simulink model "Engine_MvMdl_Ptbs_V1"  (R2018a)
settings: Solver=VariableStepAuto  StartTime=0.0  StopTime=660  FixedStep=0.001  EnableMultiTasking=on
PreLoadFcn:
  | Engine_MapMdl_Ptbs_V1_BusInfo
model workspace (MAT data in the model file):
  DiffRatio = 3.421
  EV_current = 200
  EV_motion = [20 4 0.8]
  EV_sf = 2000
  EngDriveRatio = 0.813008130081
  Fs = 0
  Fv = 0.0025
  Jcomp = 0.0227
  Jengine = 0.22
  Ki = 251.3274
  Kisa = 346.6583
  Kp_d = 0.47149
  Kp_q = 0.52125
  Ksa = 85.4316
  Ksf = 1996.2651
  Ld = 0.0003752
  Ldq = [0.0003752 0.0004148]
  Lq = 0.0004148
  Mechanical = [0.0227 0.0025 0]
  MotGbRatio = 1
  P = 4
  PolePairs = 4
  RWheel = 0.3
  Rs = 0.2
  T_max = 120
  T_mtpa = [0 13.3131834767 26.6278836885 39.9456159322 53.2678926341 66.5962219318 79.9321062746 93.277041051 106.632513247 120.000000141]
  b_axle = Simulink.Parameter
  b_axle.Value = 10
  b_axle.DataType = 'auto'
  b_axle.Dimensions = [1 1]
  b_driveshaft = Simulink.Parameter
  b_driveshaft.Value = 10
  b_driveshaft.DataType = 'auto'
  b_driveshaft.Dimensions = [1 1]
  ba = 3.4029
  id_mtpa = [0 -0.114523352646 -0.457989076459 -1.03008464374 -1.83029075221 -2.85788367342 -4.11193850568 -5.59133329791 -7.29475400168 -9.22070020138]
  idq0 = [0 0]
  idq_limits = [-9.220699542 166.993501392 167.247872355]
  iq_mtpa = [0 18.5827440345 37.1633719111 55.7397734896 74.3098506185 92.871523015 111.422734008 129.961456105 148.485696337 166.993501356]
  k_axle = Simulink.Parameter
  k_axle.Value = 5000
  k_axle.DataType = 'auto'
  k_axle.Dimensions = [1 1]
  k_driveshaft = Simulink.Parameter
  k_driveshaft.Value = 1000
  k_driveshaft.DataType = 'auto'
  k_driveshaft.Dimensions = [1 1]
  lambda_pm = 0.1194
  mechanical = [0.0227 0.0025 0]
  mot.max_trq = 307
  mot.max_pwr = 124
  mot.spd = [0 500 1000 1500 2000 2500 3000 3500 3857.04487493 4000 4500 5000 5500 6000 6500 7000 7500 8000 8500 9000 9500 10000 10500 11000 11500 12000 12500]
  mot.trq = [307 307 307 307 307 307 307 307 307 296.028194151 263.136172579 236.822555321 215.29323211 197.352129434 182.171196401 169.158968086 157.881703547 148.014097075 139.307385483 131.568086289 124.643450169 118.41127766 112.772645391 107.646616055 102.9663284 98.676064717 94.7290221283]
  mot.trq_cp = [296.028194151 263.136172579 236.822555321 215.29323211 197.352129434 182.171196401 169.158968086 157.881703547 148.014097075 139.307385483 131.568086289 124.643450169 118.41127766 112.772645391 107.646616055 102.9663284 98.676064717 94.7290221283]
  mot.J = 0.02
  mot.damp = 0.0001
  mot.Tc = 0.0267
  mot.map.spdindex = [0 1000 2000 3000 3857 4000 5000 6000 7000 8000 9000 10000 11000 12000 12584]
  mot.map.trqindex = [10 25 50 75 100 125 150 175 200 225 250 275 300 307]
  mot.map.eff = [84  90  90  90  90  90  90  90  90  90  90  90  90  90  90; 84  90  93  95  95  95  96  95  95  95  95  93  93  93  93; 84  90  93  95  95  95  96  95  96  95  95  95  95  93  93; 84  90  93  95  95  95  96  96  96  95  95  95  95  93  93; 84  90  93  95  95  95  96  96  96  95  95  93  93  93  90; 84  88  90  93  93  95  95  96  95  95  95  93  93  93  90; 84  88  90  90  90  93  95  95  95  93  93  93  93  93  90; 84  88  90  90  90  90  93  93  93  93  93  93  93  93  90; 84  84  88  90  90  90  93  93  93  93  93  93  93  93  90; 84  84  88  90  90  90  90  93  93  93  93  93  93  93  90; 84  84  84  90  90  90  90  93  93  93  93  93  93  93  90; 84  84  84  88  90  90  90  93  93  93  93  93  93  93  90; 84  84  84  88  88  88  90  93  93  93  93  93  93  93  90; 84  84  84  88  88  88  90  93  93  93  93  93  93  93  90]
  mot.m = 30
  mot.Cp = 200
  omega_init = 0
  theta_init = 0
  wc_shaft = Simulink.Parameter
  wc_shaft.Value = 0.1
  wc_shaft.DataType = 'auto'
  wc_shaft.Dimensions = [1 1]
libraries: autolibsharedmappedengines x1
(part 1 of 3)
Description:
  | Ver1 ：
  | ブレーキモデル組み込み前に、Tireブロックから車輪速を出力できるように
  | Simscapeブロック変更したものを組み込み動作確認
  | 
  | Ver2　：
  | ブレーキモデルを組み込み。シミュレーション時間大のためソルバを
  | ode15s -> ode23tに変更して動作確認。ＯＫ
  | 
  | 
  | Ver3 ：
  | センサ（相当）信号と制御信号を整理、ただし、ブレーキモデルはコントローラ込で
  | ＰＴモデル内のまま
  | 
  | Ver4：
  | ブレーキモデル内のデータログ関連のブロックを削除し、シミュレーション時間を
  | 短縮できたので、ソルバはode15sのままにしておく。
  | DriverSubsytem追加（中身は、Signla Builderのまま）
  | 
  | Ver5：
  | Coolingモデルの追加。信号の接続はSimulink信号。
  | 
  | Ver6：
  | 暫定で、Coolingモデルの水温を読み込んで、エンジンフリクションを変化させる。
  | ただし、フリクションは0に設定し、エンジン出力には影響なし。
  | 代数ループの影響をみるため。Simulink信号に変換したうえで接続
  | －＞動作せず
  | 
  | Ver7：
  | Simscape信号のまま接続。動作問題なし。
  | 
  | Ver10：
  | Driverモデルの組み込み、10-15modeでの走行確認。
  | ブレーキ協調コントローラがないため、ブレーキモデルへのブレーキ指示信号未接続。
  | 減速はモータのみ。
  | 
  | 
  | 
  | （今後の予定）
  | エンジンクーリングモデルの追加、エンジンモデル入れ替え
  | HEVシステムの組み替え
  | Inverterモデルの接続検討
settings Model: Creator=1442442  LastModifiedBy=nishito
settings SolverCC: MaxOrder=2  ZeroCrossControl=DisableAll
settings DataIOCC: SaveFormat=Array  SignalLoggingSaveFormat=ModelDataLogs  SaveOutput=off  SignalLogging=off  DSMLogging=off  SaveTime=off
settings OptimizationCC: ExpressionDepthLimit=2147483647  LifeSpan=inf
settings DebuggingCC: AlgebraicLoopMsg=error  FcnCallInpInsideContextMsg=warning  StateNameClashWarn=warning  SFUnexpectedBacktrackingDiag=warning  SFNoUnconditionalDefaultTransitionDiag=warning  SFExecutionAtInitializationDiag=none
settings HardwareCC: ProdBitPerPointer=32  ProdBitPerSizeT=32  ProdBitPerPtrDiffT=32  ProdLargestAtomicFloat=None  ProdIntDivRoundTo=Undefined  ProdEndianess=Unspecified  ProdWordSize=32  ProdHWDeviceType=32-bit Generic
settings ModelReferenceCC: UpdateModelReferenceTargets=IfOutOfDate  PropagateSignalLabelsOutOfModel=off
settings CodeAppCC: StateflowObjectComments=on
settings GRTTargetCC: TargetLangStandard=C89/C90 (ANSI)  GeneratePreprocessorConditionals=Disable all  CombineOutputUpdateFcns=off  GRTInterface=on
settings ConfigComp: CovMetricSettings=dw  CovHtmlReporting=on  CovSaveCumulativeToWorkspaceVar=on  CovSaveSingleToWorkspaceVar=on  CovExternalEMLEnable=off  CovSFcnEnable=off
settings SimscapeCC: SimscapeNormalizeSystem=off  SimscapeLogSimulationStatistics=on  SimscapeLogOpenViewer=on  SimscapeLogLimitData=off

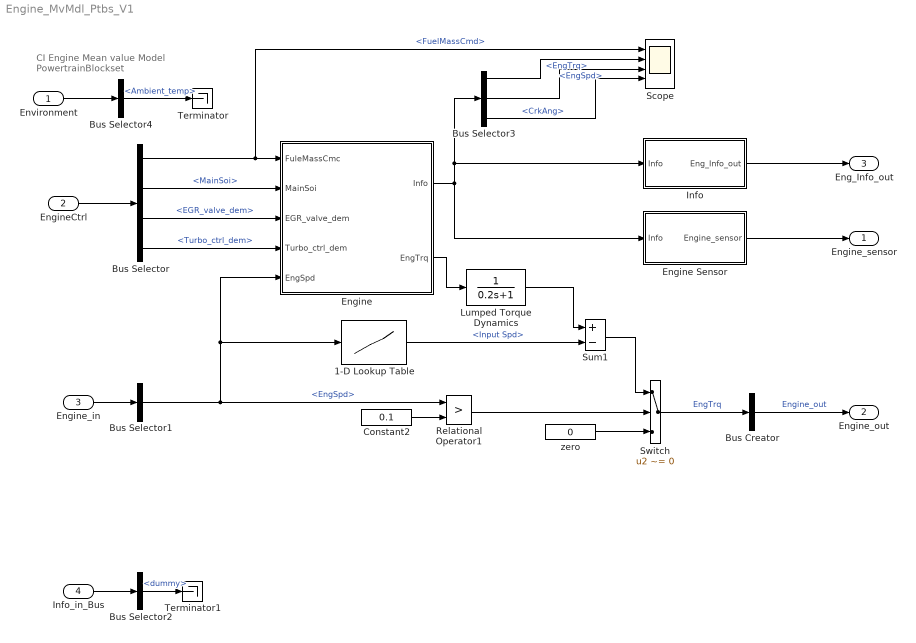
== system Engine_MvMdl_Ptbs_V1 ==
  note: CI Engine Mean value Model
      | PowertrainBlockset
  Environment : Inport  OutDataTypeStr=Bus: Environment_Bus
      settings: AttributesFormatString=%<OutDataTypeStr>
  EngineCtrl : Inport  Port=2  OutDataTypeStr=Bus: EngineCtrl_Bus
      settings: AttributesFormatString=%<OutDataTypeStr>
  Engine_in : Inport  Port=3  OutDataTypeStr=Bus: Engine_in_Bus
      settings: AttributesFormatString=%<OutDataTypeStr>
  Info_in_Bus : Inport  Port=4  OutDataTypeStr=Bus: Eng_Info_in_Bus
      settings: AttributesFormatString=%<OutDataTypeStr>
  1-D Lookup Table : Lookup_n-D  NumberOfTableDimensions=1  BreakpointsForDimension1=[0 100 200 300 400]  Table=[0 5 10 20 40]  ExtrapMethod=Clip  InternalRulePriority=Speed  RndMeth=Simplest  InputSameDT=on
  Bus Creator : BusCreator  Inputs=1  OutDataTypeStr=Bus: Engine_out_Bus
      settings: AttributesFormatString=%<OutDataTypeStr>
  Bus Selector : BusSelector  OutputSignals=FuelMassCmd,MainSoi,EGR_valve_dem,Turbo_ctrl_dem
  Bus Selector1 : BusSelector  OutputSignals=EngSpd
  Bus Selector2 : BusSelector  OutputSignals=dummy
  Bus Selector3 : BusSelector  OutputSignals=EngTrq,EngSpd,CrkAng
  Bus Selector4 : BusSelector  OutputSignals=Ambient_temp
  Constant2 : Constant  Value=0.1
  Engine : Subsystem
  Engine Sensor : Subsystem
  Info : Subsystem
  Lumped Torque Dynamics : TransferFcn  Denominator=[0.2 1]
  Relational Operator1 : RelationalOperator  Operator=>  OutDataTypeStr=boolean  RndMeth=Nearest
  Scope : Scope  NumInputPorts=4
  Sum1 : Sum  Inputs=+-
  Switch : Switch  Criteria=u2 ~= 0  Threshold=0.5  SaturateOnIntegerOverflow=on
      settings: AttributesFormatString=<%<Criteria>>
  Terminator : Terminator
  Terminator1 : Terminator
  zero : Constant  Value=0
  Engine_sensor : Outport  OutDataTypeStr=Bus: Engine_sensor_Bus
      settings: AttributesFormatString=%<OutDataTypeStr>
  Engine_out : Outport  Port=2  OutDataTypeStr=Bus: Engine_out_Bus
      settings: AttributesFormatString=%<OutDataTypeStr>
  Eng_Info_out : Outport  Port=3  OutDataTypeStr=Bus: Eng_Info_out_Bus
      settings: AttributesFormatString=%<OutDataTypeStr>
  wires:
  Bus Selector1/1 -> Engine/5(EngSpd), 1-D Lookup Table/1, Relational Operator1/1  "<EngSpd>"
  Sum1/1 -> Switch/1
  Bus Selector3/1 -> Scope/2  "<EngTrq>"
  EngineCtrl/1 -> Bus Selector/1
  1-D Lookup Table/1 -> Sum1/2  "<Input Spd>"
  Relational Operator1/1 -> Switch/2
  Constant2/1 -> Relational Operator1/2
  Engine Sensor/1(Engine_sensor) -> Engine_sensor/1
  Lumped Torque Dynamics/1 -> Sum1/1
  Bus Selector3/2 -> Scope/3  "<EngSpd>"
  Bus Selector/1 -> Engine/1(FuleMassCmc), Scope/1  "<FuelMassCmd>"
  Bus Selector3/3 -> Scope/4  "<CrkAng>"
  Switch/1 -> Bus Creator/1  "EngTrq"
  zero/1 -> Switch/3
  Environment/1 -> Bus Selector4/1
  Info_in_Bus/1 -> Bus Selector2/1
  Engine_in/1 -> Bus Selector1/1
  Bus Selector2/1 -> Terminator1/1  "<dummy>"
  Bus Selector4/1 -> Terminator/1  "<Ambient_temp>"
  Info/1(Eng_Info_out) -> Eng_Info_out/1
  Bus Creator/1 -> Engine_out/1  "Engine_out"
  Engine/1(Info) -> Bus Selector3/1, Info/1(Info), Engine Sensor/1(Info)
  Engine/2(EngTrq) -> Lumped Torque Dynamics/1
  Bus Selector/2 -> Engine/2(MainSoi)  "<MainSoi>"
  Bus Selector/3 -> Engine/3(EGR_valve_dem)  "<EGR_valve_dem>"
  Bus Selector/4 -> Engine/4(Turbo_ctrl_dem)  "<Turbo_ctrl_dem>"
